simulink model "Number_8"  (R2023b)
settings: Solver=VariableStepAuto  StartTime=0.0  StopTime=20  RelTol=1e-3
values from neighbouring files (symbols this model uses):
  G_den8 = [1 3 5 7 9 1]    [Number_7_8.m]
  G_num8 = [10 8 6 4 2]    [Number_7_8.m]
settings Model: Creator=Mariven Amurao  LastModifiedBy=Mariven Amurao

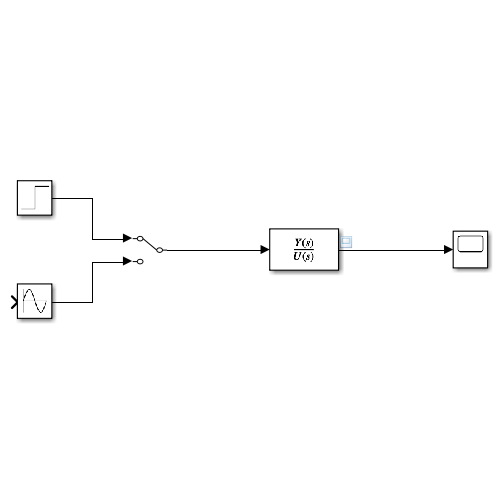
[thumbnail: Simulink's stored preview of the top-level diagram]
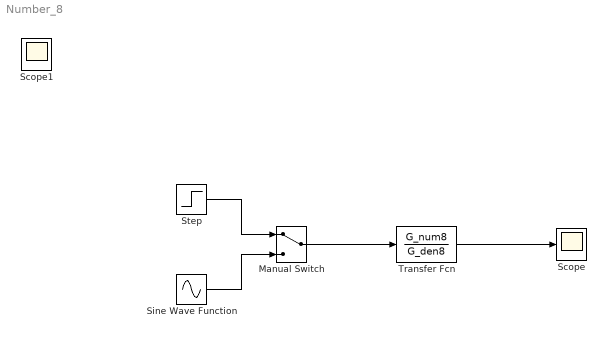
== system Number_8 ==
  Manual Switch : ManualSwitch
  Scope : Scope
  Sine Wave Function : Sin  TimeSource=Use external signal  SampleTime=0
  Step : Step  SampleTime=0
  Transfer Fcn : TransferFcn  Numerator=G_num8  Denominator=G_den8
  Scope1 : Scope
  wires:
  Transfer Fcn/1 -> Scope/1
  Manual Switch/1 -> Transfer Fcn/1
  Step/1 -> Manual Switch/1
  Sine Wave Function/1 -> Manual Switch/2
